simulink model "untitled"  (Simulink 7.5)
settings: Solver=ode45  StartTime=0.0  StopTime=10.0  FixedStep=0.01  RelTol=1e-3
undefined symbols (not defined in the file): B, J, k_m, l, L, m, R
settings Model: Creator=jorgesofrony  LastModifiedBy=jorgesofrony
settings HardwareCC: ProdBitPerInt=16  ProdIntDivRoundTo=Zero  ProdEndianess=LittleEndian  ProdWordSize=16  ProdHWDeviceType=Texas Instruments->MSP430

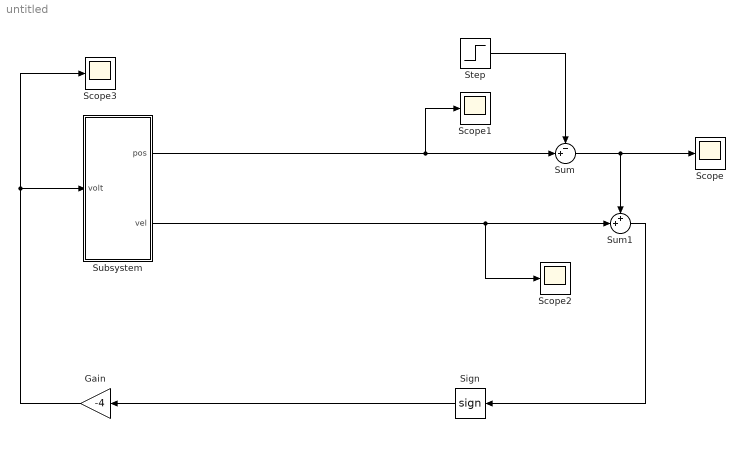
== system untitled ==
  Gain : Gain  Gain=-4  ParameterDataType=fixdt(1, 16)  ParameterScaling=2^0  OutDataType=fixdt(1, 16)  OutScaling=2^0
  Scope{,1..3} (4 alike) : Scope
      Scope settings: YMin=-1.1  YMax=0
      Scope1 settings: YMin=-0.1  YMax=1
      Scope2 settings: YMin=-1.3e-06  YMax=-7.5e-07  SaveName=ScopeData2
      Scope3 settings: YMin=-0.1  YMax=1  SaveName=ScopeData3
  Sign : Signum  ZeroCross=off
  Step : Step  SampleTime=0
  Subsystem : Subsystem
  Sum : Sum  Inputs=-+|  OutDataType=fixdt(1, 16)  OutScaling=2^0
  Sum1 : Sum  Inputs=++|  OutDataType=fixdt(1, 16)  OutScaling=2^0
  wires:
  Subsystem/2(vel) -> Scope2/1, Sum1/2
  Sign/1 -> Gain/1
  Gain/1 -> Subsystem/1(volt), Scope3/1
  Step/1 -> Sum/1
  Subsystem/1(pos) -> Scope1/1, Sum/2
  Sum/1 -> Sum1/1, Scope/1
  Sum1/1 -> Sign/1

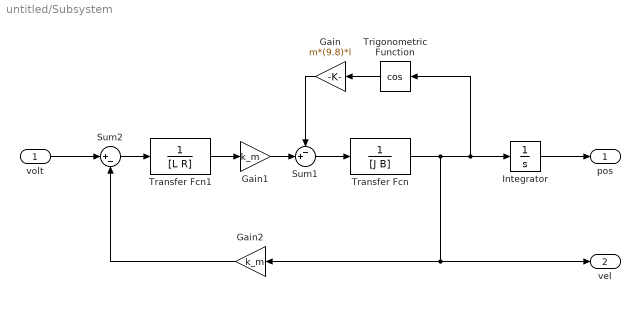
== system untitled/Subsystem ==
  volt : Inport
  Gain : Gain  Gain=m*(9.8)*l  ParameterDataType=fixdt(1, 16)  ParameterScaling=2^0  OutDataType=fixdt(1, 16)  OutScaling=2^0
  Gain1 : Gain  Gain=k_m  ParameterDataType=fixdt(1, 16)  ParameterScaling=2^0  OutDataType=fixdt(1, 16)  OutScaling=2^0
  Gain2 : Gain  Gain=k_m  ParameterDataType=fixdt(1, 16)  ParameterScaling=2^0  OutDataType=fixdt(1, 16)  OutScaling=2^0
  Integrator : Integrator  ZeroCross=off
  Sum1 : Sum  Inputs=-+|  OutDataType=fixdt(1, 16)  OutScaling=2^0
  Sum2 : Sum  Inputs=|+-  OutDataType=fixdt(1, 16)  OutScaling=2^0
  Transfer Fcn : TransferFcn  Denominator=[J B]
  Transfer Fcn1 : TransferFcn  Denominator=[L R]
  Trigonometric Function : Trigonometry  Operator=cos
  pos : Outport
  vel : Outport  Port=2
  wires:
  Transfer Fcn/1 -> Trigonometric Function/1, Integrator/1, Gain2/1, vel/1
  Sum1/1 -> Transfer Fcn/1
  Transfer Fcn1/1 -> Gain1/1
  Sum2/1 -> Transfer Fcn1/1
  Gain/1 -> Sum1/1
  volt/1 -> Sum2/1
  Trigonometric Function/1 -> Gain/1
  Gain1/1 -> Sum1/2
  Gain2/1 -> Sum2/2
  Integrator/1 -> pos/1
